simulink model "road"  (R2018a)
settings: Solver=VariableStepAuto  StartTime=0.0  StopTime=10.0  RelTol=1e-3
libraries: simulink x4
settings Model: Creator=Saurabh Suman  LastModifiedBy=Saurabh Suman

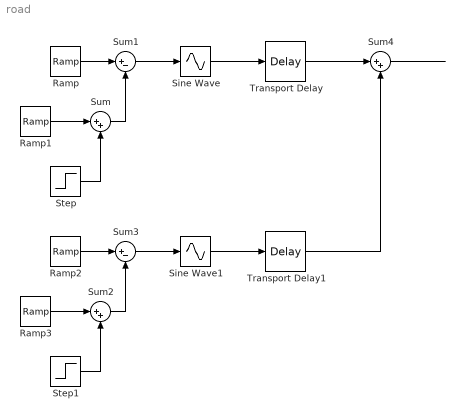
== system road ==
  Ramp : simulink/Sources/Ramp  slope=1  start=0  InitialOutput=0
  Ramp1 : simulink/Sources/Ramp  slope=1  start=1.75  InitialOutput=0
  Ramp2 : simulink/Sources/Ramp  slope=1  start=0  InitialOutput=0
  Ramp3 : simulink/Sources/Ramp  slope=1  start=1.75  InitialOutput=0
  Sine Wave : Sin  TimeSource=Use external signal  Amplitude=0.08  Frequency=1.7953  SampleTime=0
  Sine Wave1 : Sin  TimeSource=Use external signal  Amplitude=0.05  Frequency=1.7953  SampleTime=0
  Step : Step  Time=1.75  After=1.75  SampleTime=0
  Step1 : Step  Time=1.75  After=1.75  SampleTime=0
  Sum : Sum  Inputs=|++
  Sum1 : Sum  Inputs=|+-
  Sum2 : Sum  Inputs=|++
  Sum3 : Sum  Inputs=|+-
  Sum4 : Sum  Inputs=|++
  Transport Delay : TransportDelay  DelayTime=10
  Transport Delay1 : TransportDelay  DelayTime=30
  wires:
  Ramp/1 -> Sum1/1
  Ramp1/1 -> Sum/1
  Sum/1 -> Sum1/2
  Step/1 -> Sum/2
  Sine Wave/1 -> Transport Delay/1
  Sum1/1 -> Sine Wave/1
  Sum3/1 -> Sine Wave1/1
  Step1/1 -> Sum2/2
  Ramp2/1 -> Sum3/1
  Sum2/1 -> Sum3/2
  Sine Wave1/1 -> Transport Delay1/1
  Ramp3/1 -> Sum2/1
  Transport Delay/1 -> Sum4/1
  Transport Delay1/1 -> Sum4/2
  Sum4/1 -> ?
